simulink model "MVS_Dynamic_Trigger_Two_Layers_RA"  (R2024a)
settings: Solver=ode5  StartTime=0.0  StopTime=180  FixedStep=0.01  RelTol=1e-3
(part 4 of 4)

== matlab function MVS_Dynamic_Trigger_Two_Layers_RA/High-Level Agent 5/Trajectory Planner/Input compensator ==
  data: u_i_track input; u_i_restrict input; u_i output; delta_low_norm input
function u_i  = input_compensator(u_i_track, u_i_restrict, delta_low_norm)

%% Basic parameters
r_2 = 0.5;
r_3 = 0.8;

%% Calculate the actual control input
scenario = 1;

switch scenario
    case 1
        if delta_low_norm < r_2
            u_i = u_i_track;
        elseif delta_low_norm >= r_2 && delta_low_norm < r_3
            u_i = (r_3 - delta_low_norm)/(r_3 - r_2) * u_i_track + (delta_low_norm - r_2)/(r_3 - r_2) * u_i_restrict;
        else
            u_i = u_i_restrict;
        end

    case 2
        u_i = u_i_track;
end

end

== matlab function MVS_Dynamic_Trigger_Two_Layers_RA/High-Level Agent 5/Trajectory Planner/State select ==
  data: states_high input; v_i output; states_low input; delta_x_tilde output; delta_v_tilde output; a_d output
function [v_i, delta_x_tilde, delta_v_tilde, a_d] = state_select(states_high, states_low)

delta_x_tilde = states_high(1:3) - states_low(1:3);
delta_v_tilde = states_high(4:6) - states_low(4:6);
a_d = states_low(7:9);
v_i = states_high(4:6);

end

== matlab function MVS_Dynamic_Trigger_Two_Layers_RA/Communication Preparation 1/Event Tigger Mechanism/Event trigger ==
  data: time input; E_norm output; trigger_flag output; info_trigger output; delta_xi_now input; beta_i output; delta_vi_now input; e_tilde input; info_prev input; beta_i_prev input
function [E_norm, trigger_flag, info_trigger, beta_i] = event_trigger_commu(time, delta_xi_now, delta_vi_now, e_tilde, info_prev, beta_i_prev)

dimension = 3;

commu_step = 0.01;
step_size = 0.01;

if mod(time,commu_step) == 0

    E_xi = delta_xi_now - info_prev(dimension * 0 + 1 : dimension * 1);
    E_vi = delta_vi_now - info_prev(dimension * 1 + 1 : dimension * 2);
    trigger_flag = 0;
    info_trigger = info_prev;
    
    Q_max = 3.0;
    A_tilde = 2.5;
    P_min = 0.4;
    Lambda_min = 2;
    C_i = 2* eye(3);
    Lambda_i = 2* eye(3);
    rho_2 = 0.6;
    rho_3 = 2;
    alpha_1 = 1;
    
    gamma_2 = 0.5;
    
    F_2 = norm(Q_max * A_tilde * C_i * E_vi)^2/2 + norm(Q_max * A_tilde * C_i * Lambda_i * E_xi)^2/2 + 5 * rho_2 * P_min * Lambda_min * A_tilde^2 * norm(E_xi)^2 - 3 * rho_2 * P_min * Lambda_min * norm(e_tilde)^2/4;
    
    % Trigger check
    if F_2 - gamma_2 * beta_i_prev >=0
        trigger_flag = 1;
        F_2 = - 3 * rho_2 * P_min * Lambda_min * norm(e_tilde)^2/4;
        info_trigger = [delta_xi_now; delta_vi_now];
    end
    
    % If we abandon the event triggered scheme
    % info_trigger = [delta_xi_now; delta_vi_now];
    
    E_norm = norm(info_trigger - [delta_xi_now; delta_vi_now]);
    
    beta_i_dot = - alpha_1 * beta_i_prev - F_2 + rho_3;
    
    beta_i = beta_i_prev + beta_i_dot * step_size;

else
    info_trigger = info_prev;
    E_norm = norm(info_trigger - [delta_xi_now; delta_vi_now]);
    trigger_flag = 0;
    beta_i = beta_i_prev;
end

end

== matlab function MVS_Dynamic_Trigger_Two_Layers_RA/High-Level Agent 6/Trajectory Planner/Cooperative tracking/Nominal sliding mode controller ==
  data: u_i_slide output; e_tilde_xi input; e_tilde_vi input; delta_xi input; delta_vi input; acl_ref_agent input
function u_i_slide = nominal_sliding_controller(e_tilde_xi, e_tilde_vi, delta_xi, delta_vi, acl_ref_agent)

%% This is the nominal sliding mode controller for precise reference tracking

%% Basic parameters
C_i = 2 * eye(3);
Lambda_i = 2 * eye(3);

%% Controller
% Control input
S_tilde_i = e_tilde_vi + Lambda_i * e_tilde_xi;

u_i_slide = - C_i * S_tilde_i - Lambda_i * delta_vi - delta_xi + acl_ref_agent;

end

== matlab function MVS_Dynamic_Trigger_Two_Layers_RA/High-Level Agent 6/Trajectory Planner/Input compensator ==
  data: u_i_track input; u_i_restrict input; u_i output; delta_low_norm input
function u_i  = input_compensator(u_i_track, u_i_restrict, delta_low_norm)

%% Basic parameters
r_2 = 0.5;
r_3 = 0.8;

%% Calculate the actual control input
scenario = 1;

switch scenario
    case 1
        if delta_low_norm < r_2
            u_i = u_i_track;
        elseif delta_low_norm >= r_2 && delta_low_norm < r_3
            u_i = (r_3 - delta_low_norm)/(r_3 - r_2) * u_i_track + (delta_low_norm - r_2)/(r_3 - r_2) * u_i_restrict;
        else
            u_i = u_i_restrict;
        end

    case 2
        u_i = u_i_track;
end

end

== matlab function MVS_Dynamic_Trigger_Two_Layers_RA/High-Level Agent 6/Trajectory Planner/State select ==
  data: states_high input; v_i output; states_low input; delta_x_tilde output; delta_v_tilde output; a_d output
function [v_i, delta_x_tilde, delta_v_tilde, a_d] = state_select(states_high, states_low)

delta_x_tilde = states_high(1:3) - states_low(1:3);
delta_v_tilde = states_high(4:6) - states_low(4:6);
a_d = states_low(7:9);
v_i = states_high(4:6);

end

== matlab function MVS_Dynamic_Trigger_Two_Layers_RA/UGV 1/Angle adjustment ==
  data: state input; state output
function state = ang_adjust(state)

while abs(state(3)) > pi
    state(3) = state(3) - sign(state(3)) * 2 * pi;
end

end

== matlab function MVS_Dynamic_Trigger_Two_Layers_RA/UGV 1/Bike kinematics ==
  data: input input; t input; velocity output; prev_state input
function velocity = bike_kinematics(input, t, prev_state)

%% Input = [v_r, tan(delta)]
% v_r: speed of the rear wheel
% delta: steering angle of the front wheel

phi = prev_state(3);

l_r = 1.4;  % Distance between the center and the rear wheel
l_f = 1.4;  % Distance between the center and the front wheel
beta = atan(l_r/(l_r + l_f) * input(2));

%% Uncertainty
if t > 5 && t <= 20
    x_dot = max( min(input(1)/cos(beta) * cos(beta + phi), 2.7), -2.7 );
    y_dot = max( min(input(1)/cos(beta) * sin(beta + phi), 1.35), -1.35 );
    phi_dot = input(1)/(l_r + l_f) * input(2) - 0.1;
else
    x_dot = input(1)/cos(beta) * cos(beta + phi);
    y_dot = input(1)/cos(beta) * sin(beta + phi);
    phi_dot = input(1)/(l_r + l_f) * input(2);
end

% w_i = zeros(3,1);

velocity = [x_dot; y_dot; phi_dot];

end

== matlab function MVS_Dynamic_Trigger_Two_Layers_RA/UGV 1/Kinematics controller/Error calculation ==
  data: ref_3d input; pos_bike input; vel_rear output; tan_sigma output; pos_error_global output; pos_error_body output; t input
function [vel_rear, tan_sigma, pos_error_global, pos_error_body] = controller(ref_3d, pos_bike, t)

%% Basic parameters
vel_limit = 7;
% tan_limit = sqrt(3);
tan_limit = tan(2/9 * pi);
k_long = 2;
k_lat = 2;
l_r = 1.4;  % Distance between the center and the rear wheel
l_f = 1.4;  % Distance between the center and the front wheel

%% Vehicle yaw angle
phi_now = pos_bike(3);
ref_bike = kron(eye(2), [1,0,0;0,1,0]) * ref_3d(1:6);

%% Error calculation
pos_error_global = pos_bike(1:2) - ref_bike(1:2);
pos_error_body = [cos(phi_now), sin(phi_now); -sin(phi_now), cos(phi_now)] * pos_error_global;

%% Speed input
vel_rear = cos(phi_now) * ref_bike(3) + sin(phi_now) * ref_bike(4) - k_long * pos_error_body(1);

vel_rear = max( min(vel_rear, vel_limit), -vel_limit);

%% Angular input
tan_sigma = (cos(phi_now) * ref_bike(4) - sin(phi_now) * ref_bike(3) - k_lat *  pos_error_body(2))/(vel_rear * l_r) * (l_r + l_f);

tan_sigma = max( min(tan_sigma, tan_limit), -tan_limit);



end

== matlab function MVS_Dynamic_Trigger_Two_Layers_RA/UGV 1/MATLAB Function ==
  data: veh_pos input; low_states output; veh_vel input; veh_acc input
function low_states = info_collect(veh_pos, veh_vel, veh_acc)

low_states = kron(eye(3), diag([1,1,0])) * [veh_pos; veh_vel; veh_acc];

end

== matlab function MVS_Dynamic_Trigger_Two_Layers_RA/UGV 2/Angle adjustment ==
  data: state input; state output
function state = ang_adjust(state)

while abs(state(3)) > pi
    state(3) = state(3) - sign(state(3)) * 2 * pi;
end

end

== matlab function MVS_Dynamic_Trigger_Two_Layers_RA/UGV 2/Bike kinematics ==
  data: input input; t input; velocity output; prev_state input
function velocity = bike_kinematics(input, t, prev_state)

%% Input = [v_r, tan(delta)]
% v_r: speed of the rear wheel
% delta: steering angle of the front wheel

phi = prev_state(3);

l_r = 1.4;  % Distance between the center and the rear wheel
l_f = 1.4;  % Distance between the center and the front wheel

beta = atan(l_r/(l_r + l_f) * input(2));

%% Uncertainty
if t > 50 && t <= 70
    x_dot = max( min(input(1)/cos(beta) * cos(beta + phi) -0.1 * sin(0.5 * t) - 0.5, 2.6), -2.6 );
    y_dot = max( min(input(1)/cos(beta) * sin(beta + phi) -0.4 * cos(0.5 * t), 2.6), -2.6 );
    phi_dot = input(1)/(l_r + l_f) * input(2) - 0.1;
else
    x_dot = input(1)/cos(beta) * cos(beta + phi);
    y_dot = input(1)/cos(beta) * sin(beta + phi);
    phi_dot = input(1)/(l_r + l_f) * input(2);
end

velocity = [x_dot; y_dot; phi_dot];

end

== matlab function MVS_Dynamic_Trigger_Two_Layers_RA/UGV 2/Kinematics controller/Error calculation ==
  data: ref_3d input; pos_bike input; vel_rear output; tan_sigma output; pos_error_global output; pos_error_body output; t input
function [vel_rear, tan_sigma, pos_error_global, pos_error_body] = controller(ref_3d, pos_bike, t)

%% Basic parameters
vel_limit = 7;
% tan_limit = sqrt(3);
tan_limit = tan(2/9 * pi);
k_long = 2;
k_lat = 2;
l_r = 1.4;  % Distance between the center and the rear wheel
l_f = 1.4;  % Distance between the center and the front wheel

%% Vehicle yaw angle
phi_now = pos_bike(3);
ref_bike = kron(eye(2), [1,0,0;0,1,0]) * ref_3d(1:6);

%% Error calculation
pos_error_global = pos_bike(1:2) - ref_bike(1:2);
pos_error_body = [cos(phi_now), sin(phi_now); -sin(phi_now), cos(phi_now)] * pos_error_global;

%% 
% if t > 50 && t <= 70
%     %% Speed input
%     vel_rear = cos(phi_now) * ref_bike(3) + sin(phi_now) * ref_bike(4);
% 
%     vel_rear = max( min(vel_rear, vel_limit), -vel_limit);
% 
%     %% Angular input
%     tan_sigma = (cos(phi_now) * ref_bike(4) - sin(phi_now) * ref_bike(3) )/(vel_rear * l_r) * (l_r + l_f);
% 
%     tan_sigma = max( min(tan_sigma, tan_limit), -tan_limit);
% else
%     %% Speed input
%     vel_rear = cos(phi_now) * ref_bike(3) + sin(phi_now) * ref_bike(4) - k_long * pos_error_body(1);
% 
%     vel_rear = max( min(vel_rear, vel_limit), -vel_limit);
% 
%     %% Angular input
%     tan_sigma = (cos(phi_now) * ref_bike(4) - sin(phi_now) * ref_bike(3) - k_lat *  pos_error_body(2))/(vel_rear * l_r) * (l_r + l_f);
% 
%     tan_sigma = max( min(tan_sigma, tan_limit), -tan_limit);
% end

%% Speed input
vel_rear = cos(phi_now) * ref_bike(3) + sin(phi_now) * ref_bike(4) - k_long * pos_error_body(1);

vel_rear = max( min(vel_rear, vel_limit), -vel_limit);

%% Angular input
tan_sigma = (cos(phi_now) * ref_bike(4) - sin(phi_now) * ref_bike(3) - k_lat *  pos_error_body(2))/(vel_rear * l_r) * (l_r + l_f);

tan_sigma = max( min(tan_sigma, tan_limit), -tan_limit);


end

== matlab function MVS_Dynamic_Trigger_Two_Layers_RA/UGV 2/MATLAB Function ==
  data: veh_pos input; low_states output; veh_vel input; veh_acc input
function low_states = info_collect(veh_pos, veh_vel, veh_acc)

low_states = kron(eye(3), diag([1,1,0])) * [veh_pos; veh_vel; veh_acc];

end

== matlab function MVS_Dynamic_Trigger_Two_Layers_RA/UGV 3/Angle adjustment ==
  data: state input; state output
function state = ang_adjust(state)

while abs(state(3)) > pi
    state(3) = state(3) - sign(state(3)) * 2 * pi;
end

end

== matlab function MVS_Dynamic_Trigger_Two_Layers_RA/UGV 3/Bike kinematics ==
  data: input input; t input; velocity output; prev_state input
function velocity = bike_kinematics(input, t, prev_state)

%% Input = [v_r, tan(delta)]
% v_r: speed of the rear wheel
% delta: steering angle of the front wheel

phi = prev_state(3);

l_r = 1.4;  % Distance between the center and the rear wheel
l_f = 1.4;  % Distance between the center and the front wheel
beta = atan(l_r/(l_r + l_f) * input(2));

%% Uncertainty
if t > 20 && t <= 40
    w_i = [1.5 * sin(0.5 * t); 1.8 * cos(0.5 * t); 0.3 * sin(0.05 * t)];
else
    w_i = zeros(3,1);
end

w_i = zeros(3,1);

x_dot = input(1)/cos(beta) * cos(beta + phi);
y_dot = input(1)/cos(beta) * sin(beta + phi);
phi_dot = input(1)/(l_r + l_f) * input(2);

velocity = [x_dot; y_dot; phi_dot] + w_i;

end

== matlab function MVS_Dynamic_Trigger_Two_Layers_RA/UGV 3/Kinematics controller/Error calculation ==
  data: ref_3d input; pos_bike input; vel_rear output; tan_sigma output; pos_error_global output; pos_error_body output
function [vel_rear, tan_sigma, pos_error_global, pos_error_body] = controller(ref_3d, pos_bike)

%% Basic parameters
vel_limit = 7;
tan_limit = tan(2/9 * pi);
k_long = 2;
k_lat = 2;
l_r = 1.4;  % Distance between the center and the rear wheel
l_f = 1.4;  % Distance between the center and the front wheel

%% Vehicle yaw angle
phi_now = pos_bike(3);
ref_bike = kron(eye(2), [1,0,0;0,1,0]) * ref_3d(1:6);

%% Error calculation
pos_error_global = pos_bike(1:2) - ref_bike(1:2);
pos_error_body = [cos(phi_now), sin(phi_now); -sin(phi_now), cos(phi_now)] * pos_error_global;

%% Speed input
vel_rear = cos(phi_now) * ref_bike(3) + sin(phi_now) * ref_bike(4) - k_long * pos_error_body(1);

vel_rear = max( min(vel_rear, vel_limit), -vel_limit);

%% Angular input
tan_sigma = (cos(phi_now) * ref_bike(4) - sin(phi_now) * ref_bike(3) - k_lat *  pos_error_body(2))/(vel_rear * l_r) * (l_r + l_f);

tan_sigma = max( min(tan_sigma, tan_limit), -tan_limit);

end

== matlab function MVS_Dynamic_Trigger_Two_Layers_RA/UGV 3/MATLAB Function ==
  data: veh_pos input; low_states output; veh_vel input; veh_acc input
function low_states = info_collect(veh_pos, veh_vel, veh_acc)

low_states = kron(eye(3), diag([1,1,0])) * [veh_pos; veh_vel; veh_acc];

end

== matlab function MVS_Dynamic_Trigger_Two_Layers_RA/UGV 4/Angle adjustment ==
  data: state input; state output
function state = ang_adjust(state)

while abs(state(3)) > pi
    state(3) = state(3) - sign(state(3)) * 2 * pi;
end

end

== matlab function MVS_Dynamic_Trigger_Two_Layers_RA/Communication Preparation 3/Event Tigger Mechanism/Event trigger ==
  data: time input; E_norm output; trigger_flag output; info_trigger output; delta_xi_now input; beta_i output; delta_vi_now input; e_tilde input; info_prev input; beta_i_prev input
function [E_norm, trigger_flag, info_trigger, beta_i] = event_trigger_commu(time, delta_xi_now, delta_vi_now, e_tilde, info_prev, beta_i_prev)

dimension = 3;

commu_step = 0.01;
step_size = 0.01;

if mod(time,commu_step) == 0

    E_xi = delta_xi_now - info_prev(dimension * 0 + 1 : dimension * 1);
    E_vi = delta_vi_now - info_prev(dimension * 1 + 1 : dimension * 2);
    trigger_flag = 0;
    info_trigger = info_prev;
    
    Q_max = 3.0;
    A_tilde = 2.5;
    P_min = 0.4;
    Lambda_min = 2;
    C_i = 2* eye(3);
    Lambda_i = 2* eye(3);
    rho_2 = 0.3;
    rho_3 = 0.5;
    alpha_1 = 1;
    
    gamma_2 = 0.5;
    
    F_2 = norm(Q_max * A_tilde * C_i * E_vi)^2/2 + norm(Q_max * A_tilde * C_i * Lambda_i * E_xi)^2/2 + 5 * rho_2 * P_min * Lambda_min * A_tilde^2 * norm(E_xi)^2 - 3 * rho_2 * P_min * Lambda_min * norm(e_tilde)^2/4;
    
    % Trigger check
    if F_2 - gamma_2 * beta_i_prev >=0
        trigger_flag = 1;
        F_2 = - 3 * rho_2 * P_min * Lambda_min * norm(e_tilde)^2/4;
        info_trigger = [delta_xi_now; delta_vi_now];
    end
    
    % If we abandon the event triggered scheme
    % info_trigger = [delta_xi_now; delta_vi_now];
    
    E_norm = norm(info_trigger - [delta_xi_now; delta_vi_now]);
    
    beta_i_dot = - alpha_1 * beta_i_prev - F_2 + rho_3;
    
    beta_i = beta_i_prev + beta_i_dot * step_size;

else
    info_trigger = info_prev;
    E_norm = norm(info_trigger - [delta_xi_now; delta_vi_now]);
    trigger_flag = 0;
    beta_i = beta_i_prev;
end

end

== matlab function MVS_Dynamic_Trigger_Two_Layers_RA/UGV 4/Bike kinematics ==
  data: input input; t input; velocity output; prev_state input
function velocity = bike_kinematics(input, t, prev_state)

%% Input = [v_r, tan(delta)]
% v_r: speed of the rear wheel
% delta: steering angle of the front wheel

phi = prev_state(3);

l_r = 1.4;  % Distance between the center and the rear wheel
l_f = 1.4;  % Distance between the center and the front wheel
beta = atan(l_r/(l_r + l_f) * input(2));

%% Uncertainty
if t > 140 && t <= 155
    w_i = [0.5 * sin(0.5 * t) + 0.7; 0.4 * cos(0.8 * t) + 0.5; 0.2 * sin(0.5 * t)];
else
    w_i = zeros(3,1);
end

x_dot = input(1)/cos(beta) * cos(beta + phi);
y_dot = input(1)/cos(beta) * sin(beta + phi);
phi_dot = input(1)/(l_r + l_f) * input(2);

velocity = [x_dot; y_dot; phi_dot] + w_i;

end

== matlab function MVS_Dynamic_Trigger_Two_Layers_RA/UGV 4/Kinematics controller/Error calculation ==
  data: ref_3d input; pos_bike input; vel_rear output; tan_sigma output; pos_error_global output; pos_error_body output
function [vel_rear, tan_sigma, pos_error_global, pos_error_body] = controller(ref_3d, pos_bike)

%% Basic parameters
vel_limit = 7;
tan_limit = tan(2/9 * pi);
k_long = 2;
k_lat = 2;
l_r = 1.4;  % Distance between the center and the rear wheel
l_f = 1.4;  % Distance between the center and the front wheel

%% Vehicle yaw angle
phi_now = pos_bike(3);
ref_bike = kron(eye(2), [1,0,0;0,1,0]) * ref_3d(1:6);

%% Error calculation
pos_error_global = pos_bike(1:2) - ref_bike(1:2);
pos_error_body = [cos(phi_now), sin(phi_now); -sin(phi_now), cos(phi_now)] * pos_error_global;

%% Speed input
vel_rear = cos(phi_now) * ref_bike(3) + sin(phi_now) * ref_bike(4) - k_long * pos_error_body(1);

vel_rear = max( min(vel_rear, vel_limit), -vel_limit);

%% Angular input
tan_sigma = (cos(phi_now) * ref_bike(4) - sin(phi_now) * ref_bike(3) - k_lat *  pos_error_body(2))/(vel_rear * l_r) * (l_r + l_f);

tan_sigma = max( min(tan_sigma, tan_limit), -tan_limit);

end

== matlab function MVS_Dynamic_Trigger_Two_Layers_RA/UGV 4/MATLAB Function ==
  data: veh_pos input; low_states output; veh_vel input; veh_acc input
function low_states = info_collect(veh_pos, veh_vel, veh_acc)

low_states = kron(eye(3), diag([1,1,0])) * [veh_pos; veh_vel; veh_acc];

end

== matlab function MVS_Dynamic_Trigger_Two_Layers_RA/AAV 1/Controller/controller ==
  data: state_all input; a_di input; u_nom output; delta_xi input; delta_vi input; w_hat input
function u_nom  = controller(state_all, a_di, delta_xi, delta_vi, w_hat)

%% Reverse of the control gain matrix
K_i = 0.1 * [1;1;1];
m_i = 5;
g = 9.81;
dimension = 3;

x_i = state_all(dimension * 0 + 1: dimension * 1);
v_i = state_all(dimension * 1 + 1: dimension * 2);

f_i = -[K_i(1) * v_i(1) / m_i; K_i(2) * v_i(2) /m_i; K_i(3) * v_i(3)/ m_i + g];


%% Nominal control input
lambda_1 = eye(3);
c_1 = eye(3);

s = delta_vi + lambda_1 * delta_xi;

u_nom = - f_i - w_hat - lambda_1 * delta_vi - c_1 * s - delta_xi + a_di;

end

== matlab function MVS_Dynamic_Trigger_Two_Layers_RA/AAV 1/Plant ==
  data: x_ddot output; w_i output; state_all input; u_i input; t input
function [x_ddot, w_i] = model(state_all, u_i, t)

%% Second-order plants for robots
dimension = 3;
serial_num = 5;
v_i = state_all(dimension * 1 + 1: dimension * 2);

K_i = 0.1 * [1;1;1];
m_i = 5;
g = 9.81;

f_i = -[K_i(1) * v_i(1) / m_i; K_i(2) * v_i(2) /m_i; K_i(3) * v_i(3)/ m_i + g];

if t >= 55 && t <= 70 
    w_i = [-1 * cos(0.5 * t - serial_num * pi/2); 1 * sin(0.4 * t + serial_num * pi/3); 0.8 * sin(0.6 * t + serial_num * pi/4)];
else
    w_i = zeros(3,1);
end

x_ddot = f_i + u_i + w_i;

end

== matlab function MVS_Dynamic_Trigger_Two_Layers_RA/AAV 1/Reference_abstract ==
  data: a_di output; ref input; state_all input; delta_xi output; delta_vi output
function [a_di, delta_xi, delta_vi] = ref_obtain(ref, state_all)

%% Basic parameters

dimension = 3;

x_i = state_all(dimension * 0 + 1: dimension * 1);
v_i = state_all(dimension * 1 + 1: dimension * 2);

x_di = ref(dimension * 0 + 1: dimension * 1);
v_di = ref(dimension * 1 + 1: dimension * 2);
a_di = ref(dimension * 2 + 1: dimension * 3);

delta_xi = x_i - x_di; 
delta_vi = v_i - v_di;

end

== matlab function MVS_Dynamic_Trigger_Two_Layers_RA/AAV 2/Controller/MATLAB Function ==
  data: u_nom input; u_diff output; u_sat input
function u_diff = fcn(u_nom, u_sat)

u_diff = norm(u_nom - u_sat);

end

== matlab function MVS_Dynamic_Trigger_Two_Layers_RA/AAV 2/Controller/controller ==
  data: state_all input; a_di input; u_nom output; delta_xi input; delta_vi input; w_hat input
function u_nom  = controller(state_all, a_di, delta_xi, delta_vi, w_hat)

%% Reverse of the control gain matrix
K_i = 0.1 * [1;1;1];
m_i = 5;
g = 9.81;
dimension = 3;

x_i = state_all(dimension * 0 + 1: dimension * 1);
v_i = state_all(dimension * 1 + 1: dimension * 2);

f_i = -[K_i(1) * v_i(1) / m_i; K_i(2) * v_i(2) /m_i; K_i(3) * v_i(3)/ m_i + g];


%% Nominal control input
lambda_1 = eye(3);
c_1 = eye(3);

s = delta_vi + lambda_1 * delta_xi;

u_nom = - f_i - w_hat - lambda_1 * delta_vi - c_1 * s - delta_xi + a_di;

end
